simulink model "PE6_1_Simulink"  (R2014a)
settings: Solver=ode45  SolverMode=SingleTasking  StartTime=0.0  StopTime=0.08  MaxStep=1e-4  RelTol=1e-3
libraries: powerlib x15, powerlib_meascontrol x3
settings Model: CovMetricSettings=dwe  CovHtmlReporting=off  covSaveCumulativeToWorkspaceVar=off  CovSaveSingleToWorkspaceVar=off  CovExternalEMLEnable=on  CovSFcnEnable=on  Creator=hasee  LastModifiedBy=hasee
settings DataIOCC: LimitDataPoints=off  SaveFormat=StructureWithTime
settings DebuggingCC: MergeDetectMultiDrivingBlocksExec=error  SolverPrmCheckMsg=none  FrameProcessingCompatibilityMsg=error  SFUnexpectedBacktrackingDiag=error  SFNoUnconditionalDefaultTransitionDiag=error
settings HardwareCC: ProdBitPerPointer=64  ProdLargestAtomicFloat=Float  ProdIntDivRoundTo=Zero  ProdEndianess=LittleEndian  ProdHWDeviceType=Specified
settings ModelReferenceCC: PropagateSignalLabelsOutOfModel=on
settings GRTTargetCC: TargetLangStandard=C99 (ISO)  GeneratePreprocessorConditionals=Use local settings
settings ConfigurationSet: Description=Simscape Multibody

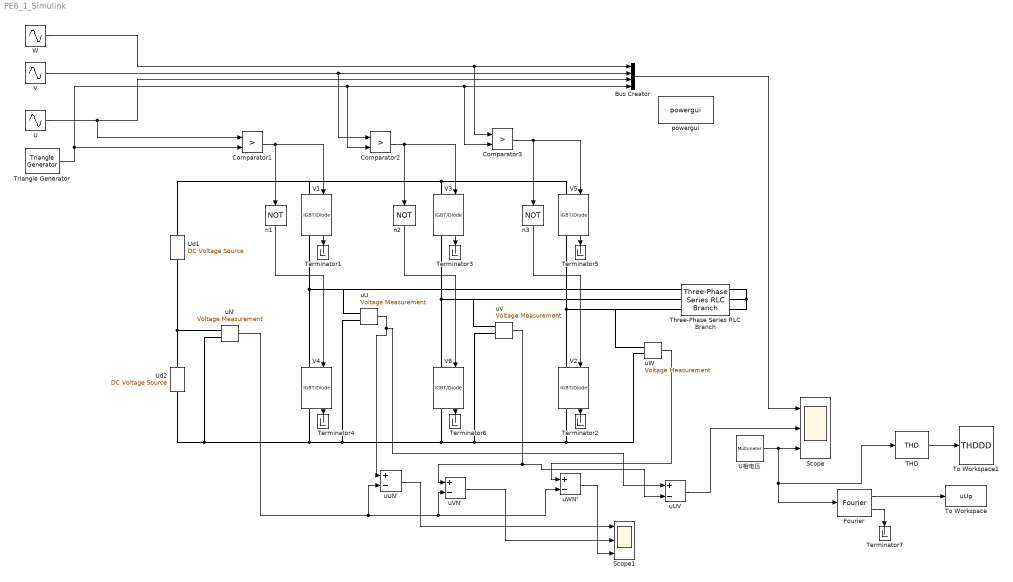
== system PE6_1_Simulink ==
  Bus Creator : BusCreator  Inputs=4
  Comparator1 : RelationalOperator  Operator=>  OutDataTypeStr=boolean
  Comparator2 : RelationalOperator  Operator=>  OutDataTypeStr=boolean
  Comparator3 : RelationalOperator  Operator=>  OutDataTypeStr=boolean
  Fourier : powerlib_meascontrol/Measurements/Fourier  Freq=50  n=[1 502 504 995 999 1502 1504 1995 1999]  InInit=[0, 0]  Ts=0
  Scope : Scope  NumInputPorts=3
      settings: TimeRange=auto  ShowLegends=on  MaxDataPoints=5000  SaveName=ScopeData  YMin=-1.25~-1187.50187~-791.66262  YMax=1.25~1187.50104~791.66091  SampleTime=-1
  Scope1 : Scope  NumInputPorts=3
      settings: TimeRange=auto  ShowLegends=on  MaxDataPoints=5000  YMin=-593.82036~-593.82019~-593.82028  YMax=593.82011~593.82036~593.82032  SampleTime=-1
  THD : powerlib_meascontrol/Measurements/THD  Freq=60  Ts=0
  Terminator{1..7} (7 alike) : Terminator
  Three-Phase Series RLC Branch : powerlib/Elements/Three-Phase Series RLC Branch  LConnTagsString=A|B|C  RConnTagsString=A|B|C  BranchType=RL  Resistance=10  Inductance=2e-3  Capacitance=1e-6  Measurements=Branch voltages
  To Workspace : ToWorkspace  VariableName=uUp  SampleTime=-1
  To Workspace1 : ToWorkspace  VariableName=THDDD  SampleTime=-1
  Triangle Generator : powerlib_meascontrol/Pulse & Signal Generators/Triangle Generator  Freq=25e3  Phase=90  Ts=0
  U : Sin  Frequency=100*pi
  Ud1 : powerlib/Electrical Sources/DC Voltage Source  Amplitude=475  Measurements=None
  Ud2 : powerlib/Electrical Sources/DC Voltage Source  Amplitude=475  Measurements=None
  U相电压 : powerlib/Measurements/Multimeter  PhasorSimulation=off  OutputType=Complex  sel=1  L=3  Gain=1  yselected={'Ub1: Three-Phase Series RLC Branch'};  PSBOutputType=1  PSBequivalent=0  AxesSetting=[0,0.1,-100,100]  Display=0  SavedBlockNames=-11
  V : Sin  Frequency=100*pi  Phase=-2/3*pi
  V{1..6} (6 alike) : powerlib/Power Electronics/IGBT//Diode  Ron=1e-3  Rs=1e5  Cs=inf  Measurements=on
  W : Sin  Frequency=100*pi  Phase=2/3*pi
  n1 : Logic  Operator=NOT  AllPortsSameDT=off  OutDataTypeStr=boolean
  n2 : Logic  Operator=NOT  AllPortsSameDT=off  OutDataTypeStr=boolean
  n3 : Logic  Operator=NOT  AllPortsSameDT=off  OutDataTypeStr=boolean
  powergui : powerlib/powergui  Priority=1  SimulationMode=Continuous  SampleTime=50e-6  frequency=60  Iterations=50  frequencyindice=0  Pbase=100e6  ErrMax=1e-4  UnitsV=kV  UnitsW=MW  buscounter=0  FunctionMessages=off  echomessages=off  EnableUseOfTLC=off  CurrentSourceSwitches=off  DisableSnubberDevices=off  DisableRonSwitches=off  DisableVfSwitches=off  DisplayEquations=off  SolverType=Tustin/Backward Euler (TBE)  Interpol=off  ExternalGateDelay=off  methode=off  Ts=100  x0status=blocks  SPID=on  SwTol=0  HookPort=off  RestoreLinks=warning  ResistiveCurrentMeasurement=off  Frange=[0:2:500]  Ylog=off  Xlog=on  ShowGrid=off  save=off  variable=ZData  structure=ScopeData  ZoomFFT=off  StartTime=0.02  cycles=1  DisplayStyle=2  fundamental=50  FreqAxis=off  MaxFrequency=10e7  frequencyindicesteady=1  RmsSteady=1  display=off
  uN' : powerlib/Measurements/Voltage Measurement  PhasorSimulation=off  OutputType=Complex  PSBequivalent=0
  uU : powerlib/Measurements/Voltage Measurement  PhasorSimulation=off  OutputType=Complex  PSBequivalent=0
  uUN' : Sum  Inputs=+-
  uUV : Sum  Inputs=+-
  uV : powerlib/Measurements/Voltage Measurement  PhasorSimulation=off  OutputType=Complex  PSBequivalent=0
  uVN' : Sum  Inputs=+-
  uW : powerlib/Measurements/Voltage Measurement  PhasorSimulation=off  OutputType=Complex  PSBequivalent=0
  uWN' : Sum  Inputs=+-
  wires:
  W/1 -> Comparator3/1, Bus Creator/1
  V/1 -> Comparator2/1, Bus Creator/2
  U/1 -> Comparator1/1, Bus Creator/3
  Triangle Generator/1 -> Comparator1/2, Comparator2/2, Comparator3/2, Bus Creator/4
  V1/1 -> Terminator1/1
  V2/1 -> Terminator2/1
  V3/1 -> Terminator3/1
  V4/1 -> Terminator4/1
  V5/1 -> Terminator5/1
  V6/1 -> Terminator6/1
  Comparator1/1 -> n1/1, V1/1
  Comparator2/1 -> n2/1, V3/1
  n1/1 -> V4/1
  n2/1 -> V6/1
  Comparator3/1 -> n3/1, V5/1
  n3/1 -> V2/1
  Bus Creator/1 -> Scope/1
  uU/1 -> uUV/1, uUN'/1
  uN'/1 -> uUN'/2, uWN'/2, uVN'/2
  uW/1 -> uWN'/1
  uV/1 -> uUV/2, uVN'/1
  U相电压/1 -> THD/1, Fourier/1, Scope/3
  uUV/1 -> Scope/2
  uUN'/1 -> Scope1/1
  uVN'/1 -> Scope1/2
  uWN'/1 -> Scope1/3
  Fourier/1 -> To Workspace/1
  Fourier/2 -> Terminator7/1
  THD/1 -> To Workspace1/1
  connections:
  Ud1/RConn1 -- V1/LConn1 -- V3/LConn1 -- V5/LConn1
  Ud1/LConn1 -- uN'/LConn1 -- Ud2/RConn1
  V1/RConn1 -- uU/LConn1 -- Three-Phase Series RLC Branch/LConn1 -- V4/LConn1
  Three-Phase Series RLC Branch/RConn3 -- Three-Phase Series RLC Branch/RConn2 -- Three-Phase Series RLC Branch/RConn1
  V3/RConn1 -- uV/LConn1 -- Three-Phase Series RLC Branch/LConn2 -- V6/LConn1
  V2/LConn1 -- uW/LConn1 -- Three-Phase Series RLC Branch/LConn3 -- V5/RConn1
  V2/RConn1 -- uW/LConn2 -- uV/LConn2 -- V6/RConn1 -- uU/LConn2 -- V4/RConn1 -- uN'/LConn2 -- Ud2/LConn1
